simulink model "AutomaticGuitarTuner"  (R2017a)
settings: Solver=FixedStepDiscrete  StartTime=0.0  StopTime=inf  FixedStep=0.0002  RelTol=1e-3  EnableMultiTasking=on
libraries: arduinolib x11
settings Model: SimulationMode=external  ExtModeTrigDuration=2  Creator=boverzat  LastModifiedBy=mgovinda
settings OptimizationCC: PassReuseOutputArgsAs=Individual arguments  MaxStackSize=64
settings DebuggingCC: ParameterTunabilityLossMsg=error
settings HardwareCC: ProdBitPerPointer=32  ProdBitPerSizeT=32  ProdBitPerPtrDiffT=32  ProdLargestAtomicInteger=Long  ProdLargestAtomicFloat=Double  ProdWordSize=32  ProdHWDeviceType=ARM Compatible->ARM Cortex
settings SFSimCC: MATLABDynamicMemAlloc=off
settings RTWCC: SystemTargetFile=ert.tlc  HardwareBoard=Arduino Due  TLCOptions=-aInlineSetEventsForThisBaseRateFcn=TLC_FALSE -aSuppressMultiTaskScheduler=TLC_FALSE -aRateBasedStepFcn=1  TemplateMakefile=ert_default_tmf  Description=Embedded Coder  GenerateReport=on  Toolchain=Arduino ARM  BuildConfiguration=Faster Runs  IncludeHyperlinkInReport=on  LaunchReport=on  GenerateTraceInfo=on  GenerateTraceReport=on  GenerateTraceReportSl=on  GenerateTraceReportSf=on  GenerateTraceReportEml=on
settings CodeAppCC: ForceParamTrailComments=on  IgnoreCustomStorageClasses=off  OperatorAnnotations=on  SimulinkDataObjDesc=on  SFDataObjDesc=on  MATLABFcnDesc=on  InsertBlockDesc=on  MATLABSourceComments=on
settings ERTTargetCC: SupportContinuousTime=on  SupportVariableSizeSignals=on

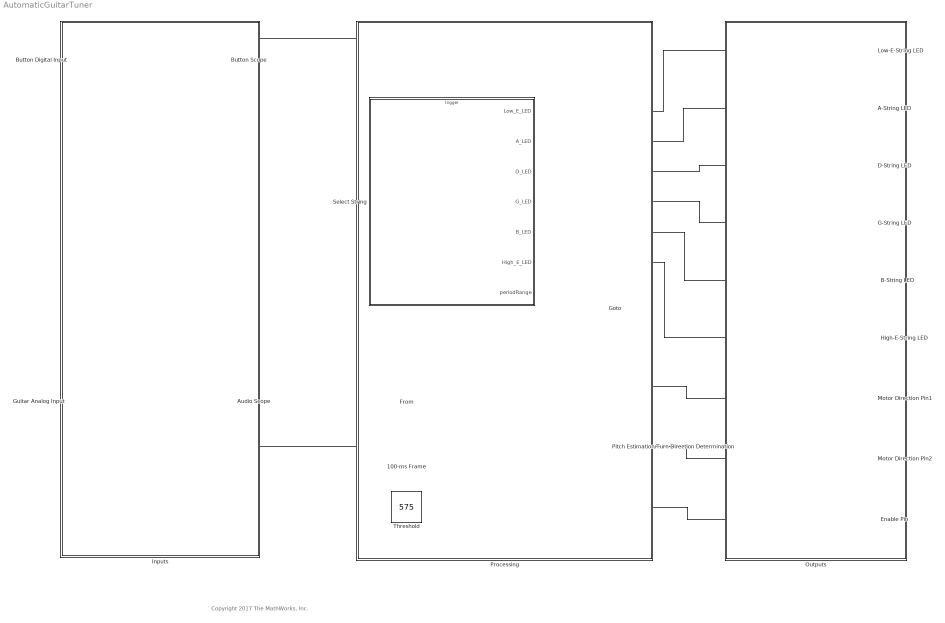
== system AutomaticGuitarTuner ==
  note: Copyright 2017 The MathWorks, Inc.
  100-ms Frame : Buffer  N=500  OutputFrames=off
  A-String LED : arduinolib/Digital Output  pinNumber=3  blockPlatform=arduino
  Audio Scope : Scope
  B-String LED : arduinolib/Digital Output  pinNumber=6  blockPlatform=arduino
  Button Digital Input : arduinolib/Digital Input  pinNumber=14  sampleTime=0.1  blockPlatform=arduino
      settings: SourceProductName=Simulink Support Package for Arduino Hardware
  Button Scope : Scope
  D-String LED : arduinolib/Digital Output  pinNumber=4  blockPlatform=arduino
  Enable Pin : arduinolib/Digital Output  pinNumber=22  blockPlatform=arduino
  G-String LED : arduinolib/Digital Output  pinNumber=5  blockPlatform=arduino
  Guitar Analog Input : arduinolib/Analog Input  pinNumber=0  sampleTime=0.0002  blockPlatform=arduino
  High-E-String LED : arduinolib/Digital Output  pinNumber=7  blockPlatform=arduino
  Inputs : Subsystem
  Low-E-String LED : arduinolib/Digital Output  pinNumber=2  blockPlatform=arduino
  Motor Direction Pin1 : arduinolib/Digital Output  pinNumber=26  blockPlatform=arduino
  Motor Direction Pin2 : arduinolib/Digital Output  pinNumber=24  blockPlatform=arduino
  Outputs : Subsystem
  Pitch Estimation/Turn Direction Determination : MATLAB Function  TreatAsAtomicUnit=on
  Processing : Subsystem
  Select String : Stateflow chart  TreatAsAtomicUnit=on
  Threshold : Constant  Value=575
  wires:
  Select String/2(A_LED) -> A-String LED/1
  Select String/3(D_LED) -> D-String LED/1
  Select String/4(G_LED) -> G-String LED/1
  Select String/5(B_LED) -> B-String LED/1
  Select String/6(High_E_LED) -> High-E-String LED/1
  Pitch Estimation/Turn Direction Determination/1(dir1) -> Motor Direction Pin1/1
  Pitch Estimation/Turn Direction Determination/2(dir2) -> Motor Direction Pin2/1
  Select String/1(Low_E_LED) -> Low-E-String LED/1
  Button Digital Input/1 -> Select String/Trigger, Button Scope/1
  Guitar Analog Input/1 -> Audio Scope/1, 100-ms Frame/1
  Pitch Estimation/Turn Direction Determination/3(enable) -> Enable Pin/1
  Threshold/1 -> Pitch Estimation/Turn Direction Determination/3(thresh)
  100-ms Frame/1 -> Pitch Estimation/Turn Direction Determination/2(frame)
  [range] -> Pitch Estimation/Turn Direction Determination/1(periodRange)
  Select String/7(periodRange) -> [range]

== system AutomaticGuitarTuner/Inputs ==

== system AutomaticGuitarTuner/Outputs ==

== system AutomaticGuitarTuner/Processing ==

== matlab function AutomaticGuitarTuner/Pitch Estimation//Turn Direction Determination ==
  data: periodRange input; frame input; dir1 output; dir2 output; thresh input; enable output
function [dir1, dir2, enable] = getTurnDirection(periodRange, frame, thresh)    
    %% Initialization 
    sampleRate = 5000;
    L = length(frame) * 0.3;
    %% Check if frame is valid based on threshold
    startOfFrame = frame(1:L);
    endOfFrame = frame((length(frame) - L):length(frame));          
    isValid = (max(startOfFrame) > thresh) && (max(endOfFrame) > thresh);
    if isValid    
        %% Determine period of waveform
        % Create Average Difference Magnitude Function (ADMF) vector
        admfLength = floor(length(frame) / 2);
        admf = zeros(admfLength,1);
        for i = 1:admfLength
            admf(i) = mean(abs(frame(1:admfLength) - frame((1 + i):(admfLength + i))));
        end
        admf = max(admf) - admf;
        %Identify peaks in ADMF vector
        peakThreshold = 0.7 * max(admf);
        admf(admf < peakThreshold) = 0;
        [~, locs] = findpeaks(admf);
        %Calculate period by averaging time between consecutive peaks
        periodInSamples = mean(diff(locs));
        periodInSeconds = periodInSamples / sampleRate;
        %Determine direction to turn tuning peg based on period and previous
        %reading
        %% Actuate motor based on determined waveform period
        if periodInSeconds < periodRange(1) && periodInSeconds > periodRange(1)/2 %Period of note is too low
            dir1 = 1;
            dir2 = 0;
            enable = 1;
        elseif periodInSeconds > periodRange(2) && periodInSeconds < periodRange(1)*2 %Period of note is too high
            dir1 = 0;
            dir2 = 1;
            enable = 1;
        elseif periodInSeconds > periodRange(1) && periodInSeconds < periodRange(2) %String is in tune
            dir1 = 0;
            dir2 = 0;
            enable = 0;
        else %Period is outside expected range and likely a false reading
            dir1 = 0;
            dir2 = 0;
            enable = 0;
        end
    else %Audio frame is not valid and pitch estimation should not be attempted
        dir1 = 0;
        dir2 = 0;
        enable = 0;
    end
end

== stateflow chart AutomaticGuitarTuner/Select String ==
  settings: executeAtInitialization=1
  state Low_E
    en: Low_E_LED = 1; periodRange = [12.065e-3, 12.205e-3];
    ex: Low_E_LED = 0;
  state A
    en: A_LED = 1; periodRange = [9.0385e-3, 9.1436e-3];
    ex: A_LED = 0;
  state D
    en: D_LED = 1; periodRange = [6.7713e-3, 6.8499e-3];
    ex: D_LED = 0;
  state G
    en: G_LED = 1; periodRange = [5.0727e-3, 5.1317e-3];
    ex: G_LED = 0;
  state B
    en: B_LED = 1; periodRange = [4.0262e-3, 4.073e-3];
    ex: B_LED = 0;
  state High_E
    en: High_E_LED = 1; periodRange = [3.0163e-3, 3.0513e-3];
    ex: High_E_LED = 0;
  (default) -> Low_E
  High_E -> Low_E : buttonPressed
  Low_E -> A : buttonPressed
  A -> D : buttonPressed
  D -> G : buttonPressed
  G -> B : buttonPressed
  B -> High_E : buttonPressed
  data: Low_E_LED output =1; A_LED output =0; D_LED output =0; G_LED output =0; B_LED output =0; High_E_LED output =0; periodRange output size=1 2
  events: buttonPressed input RISING_EDGE_EVENT
